simulink model "simulink_SetTargetPioneerVelocity"  (R2014a)
settings: Solver=ode45  StartTime=0.0  StopTime=10.0  RelTol=1e-3
settings Model: Creator=heimdall  LastModifiedBy=heimdall

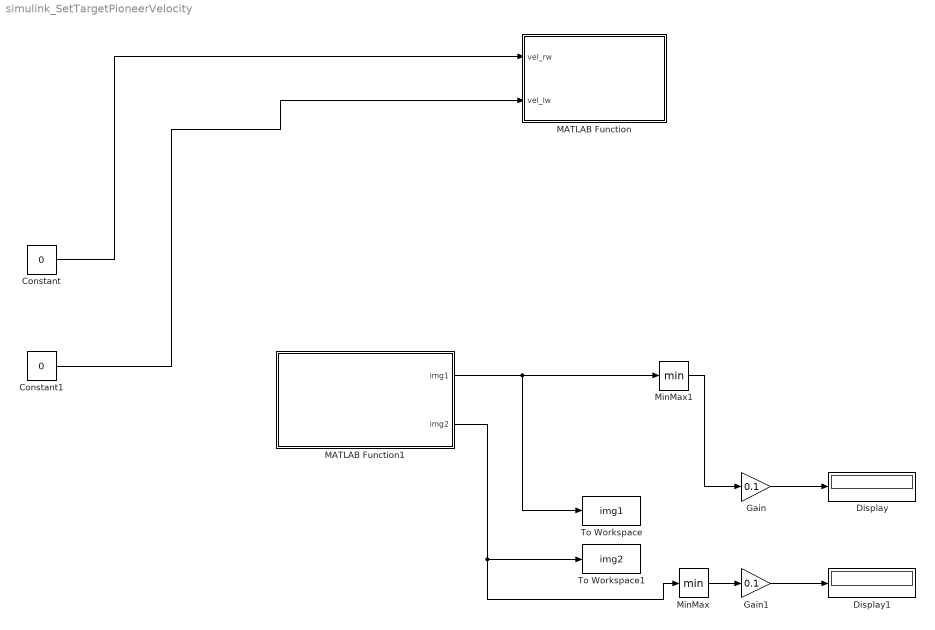
== system simulink_SetTargetPioneerVelocity ==
  Constant : Constant  Value=0  VectorParams1D=off
  Constant1 : Constant  Value=0  VectorParams1D=off
  Display : Display
  Display1 : Display
  Gain : Gain  Gain=0.1
  Gain1 : Gain  Gain=0.1
  MATLAB Function : MATLAB Function  TreatAsAtomicUnit=on
  MATLAB Function1 : MATLAB Function  TreatAsAtomicUnit=on
  MinMax : MinMax
  MinMax1 : MinMax
  To Workspace : ToWorkspace  VariableName=img1  SaveFormat=Timeseries  SampleTime=-1
  To Workspace1 : ToWorkspace  VariableName=img2  SaveFormat=Timeseries  SampleTime=-1
  wires:
  MATLAB Function1/1(img1) -> MinMax1/1, To Workspace/1
  MATLAB Function1/2(img2) -> MinMax/1, To Workspace1/1
  Constant/1 -> MATLAB Function/1(vel_rw)
  MinMax/1 -> Gain1/1
  MinMax1/1 -> Gain/1
  Constant1/1 -> MATLAB Function/2(vel_lw)
  Gain/1 -> Display/1
  Gain1/1 -> Display1/1

== matlab function simulink_SetTargetPioneerVelocity/MATLAB Function1 ==
  data: img1 output; img2 output
function [img1, img2] = simulink_getVisionSensor()
    coder.extrinsic('getVisionScanner')
    [ximg1, ximg2] = getVisionScanner();
    img1 = zeros(156,1,'double');
    img2 = zeros(256-134,1,'double');
    img1 = ximg1;
    img2 = ximg2;   
end

== matlab function simulink_SetTargetPioneerVelocity/MATLAB Function ==
  data: vel_rw input; vel_lw input
function simulink_SetTargetPioneerVelocity(vel_rw,vel_lw)
    coder.extrinsic('setTargetVelocityPioneer')
    setTargetVelocityPioneer(0,vel_rw,vel_lw)
end
